simulink model "bbcSimPID"  (R2024a)
settings: Solver=VariableStepAuto  StartTime=0.0  StopTime=4.0  FixedStep=0.0001  RelTol=1e-3
model workspace (MAT data in the model file):
  V_ref = Simulink.Parameter
  V_ref.Complexity = 'real'
  V_ref.Dimensions = [0 0]
  V_ref.DataType = 'auto'
libraries: spsSeriesRLCBranchLib x3, spsVoltageMeasurementLib x2, spsDiodeLib x1, spsMosfetLib x1, spsDCVoltageSourceLib x1, spspowerguiLib x1, spsPWMGeneratorDCDCLib x1
settings Model: Creator=krupa  LastModifiedBy=ariellevy
settings OptimizationCC: ReuseModelBlockBuffer=off
settings RTWCC: GPUComputeCapability=3.5

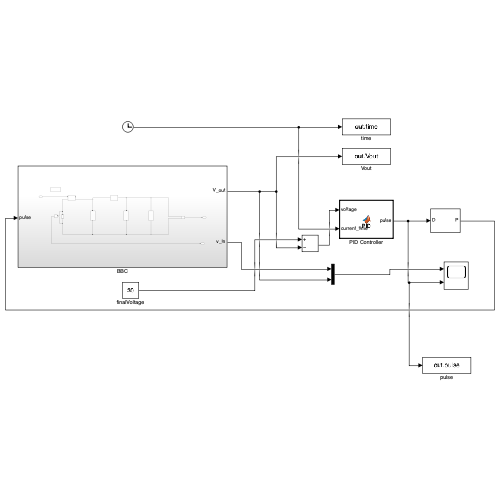
[thumbnail: Simulink's stored preview of the top-level diagram]
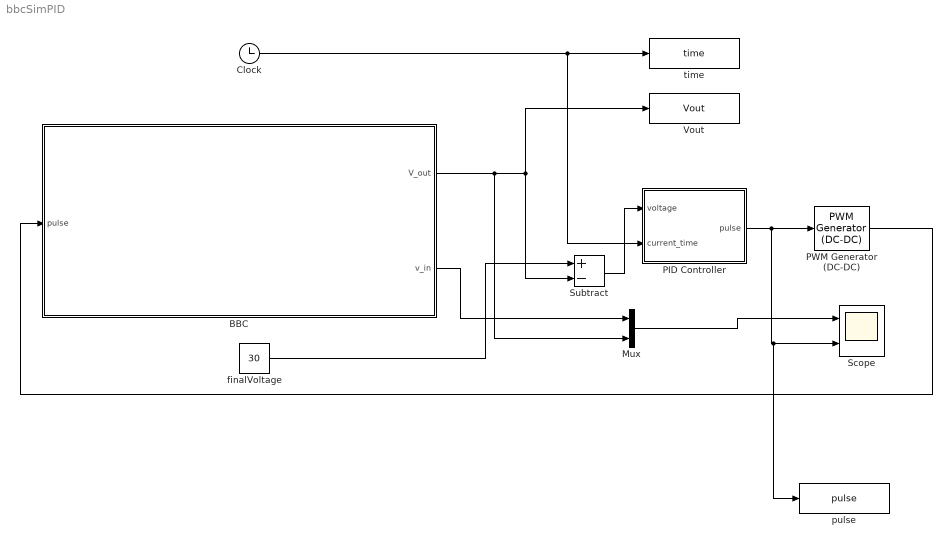
== system bbcSimPID ==
  BBC : Subsystem
  Clock : Clock
  Mux : Mux  Inputs=2
  PID Controller : MATLAB Function  TreatAsAtomicUnit=on  SystemSampleTime=0.0001
  PWM Generator (DC-DC) : spsPWMGeneratorDCDCLib/PWM Generator (DC-DC)  Fsw=10e3  Ts=0
  Scope : Scope  NumInputPorts=2
  Subtract : Sum  Inputs=+-
  Vout : ToWorkspace  VariableName=Vout  SampleTime=-1
  finalVoltage : Constant  Value=30
  pulse : ToWorkspace  VariableName=pulse  SampleTime=-1
  time : ToWorkspace  VariableName=time  SampleTime=-1
  wires:
  BBC/1(V_out) -> Mux/2, Subtract/2, Vout/1
  Clock/1 -> PID Controller/2(current_time), time/1
  PID Controller/1(pulse) -> pulse/1, Scope/2, PWM Generator (DC-DC)/1
  Subtract/1 -> PID Controller/1(voltage)
  finalVoltage/1 -> Subtract/1
  Mux/1 -> Scope/1
  BBC/2(v_in) -> Mux/1
  PWM Generator (DC-DC)/1 -> BBC/1(pulse)

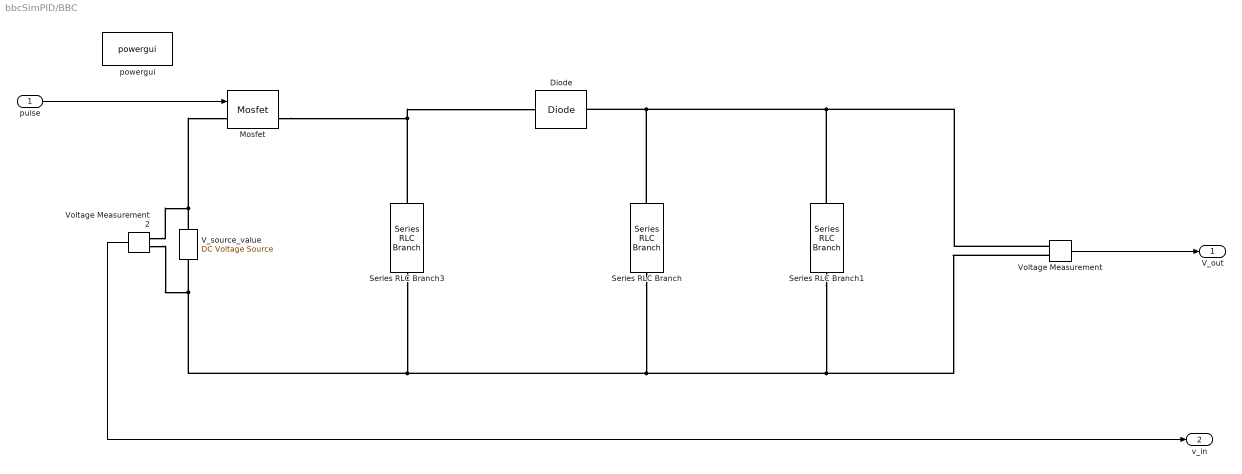
== system bbcSimPID/BBC ==
  pulse : Inport
  Diode : spsDiodeLib/Diode  Ron=0.001  Lon=0  Vf=0.8  IC=0  UseSnubber=0  Rs=500  Cs=250e-9  Measurements=off
  Mosfet : spsMosfetLib/Mosfet  Ron=0.1  Lon=0  Rd=0.01  Vfd=0  IC=0  Rs=1e5  Cs=inf  Measurements=on
  Series RLC Branch : spsSeriesRLCBranchLib/Series RLC Branch  LConnTagsString=__new0  RConnTagsString=__new0  BranchType=C  Resistance=1  Inductance=1e-3  SetiL0=off  InitialCurrent=0  Capacitance=40e-3  Setx0=off  InitialVoltage=0  Measurements=None
  Series RLC Branch1 : spsSeriesRLCBranchLib/Series RLC Branch  LConnTagsString=__new0  RConnTagsString=__new0  BranchType=R  Resistance=100  Inductance=1e-3  SetiL0=off  InitialCurrent=0  Capacitance=1e-6  Setx0=off  InitialVoltage=0  Measurements=None
  Series RLC Branch3 : spsSeriesRLCBranchLib/Series RLC Branch  LConnTagsString=__new0  RConnTagsString=__new0  BranchType=L  Resistance=1  Inductance=10e-6  SetiL0=off  InitialCurrent=0  Capacitance=1e-6  Setx0=off  InitialVoltage=0  Measurements=None
  V_source_value : spsDCVoltageSourceLib/DC Voltage Source  Amplitude=48  Measurements=Voltage
  Voltage Measurement : spsVoltageMeasurementLib/Voltage Measurement  PhasorSimulation=off  OutputType=Complex  PSBequivalent=0
  Voltage Measurement2 : spsVoltageMeasurementLib/Voltage Measurement  PhasorSimulation=off  OutputType=Complex  PSBequivalent=0
  powergui : spspowerguiLib/powergui  Priority=1  SimulationMode=Continuous  SampleTime=0.0001  frequency=60  Iterations=50  frequencyindice=0  Pbase=100e6  ErrMax=1e-4  UnitsV=kV  UnitsW=MW  buscounter=0  FunctionMessages=off  echomessages=off  EnableUseOfTLC=off  CurrentSourceSwitches=off  DisableSnubberDevices=off  DisableRonSwitches=off  DisableVfSwitches=off  DisplayEquations=off  AutomaticDiscreteSolvers=off  SolverType=Tustin/Backward Euler (TBE)  Interpol=off  ExternalGateDelay=off  methode=off  Ts=100  x0status=blocks  SPID=on  SwTol=0  HookPort=off  NonlinearTolerance=1e-4  nMaxIteration=100  ContinueOnMaxIteration=off  RestoreLinks=warning  ResistiveCurrentMeasurement=off  Frange=[0:2:500]  Ylog=off  Xlog=on  ShowGrid=off  save=off  variable=ZData  structure=0  ZoomFFT=off  StartTime=0.0  cycles=1  DisplayStyle=1  fundamental=60  FreqAxis=off  MaxFrequency=1000  frequencyindicesteady=1  RmsSteady=1  display=off
  V_out : Outport
  v_in : Outport  Port=2
  wires:
  pulse/1 -> Mosfet/1
  Voltage Measurement/1 -> V_out/1
  Voltage Measurement2/1 -> v_in/1
  connections:
  V_source_value/RConn1 -- Voltage Measurement2/LConn1 -- Mosfet/LConn1
  Mosfet/RConn1 -- Diode/RConn1 -- Series RLC Branch3/LConn1
  Voltage Measurement/LConn2 -- Series RLC Branch1/RConn1 -- Series RLC Branch/RConn1 -- Series RLC Branch3/RConn1 -- Voltage Measurement2/LConn2 -- V_source_value/LConn1
  Voltage Measurement/LConn1 -- Series RLC Branch1/LConn1 -- Series RLC Branch/LConn1 -- Diode/LConn1

== matlab function bbcSimPID/PID Controller ==
  settings: updateMethod=DISCRETE
  data: voltage input; pulse output; current_time input
function pulse = PID(voltage, current_time)

    % call extrinsic python function
    coder.extrinsic('py.PIDControllerBBC.controller_call');

    % Call Python function and return result
    pulse = coder.nullcopy(zeros(1,1)); % no clue why, but this is need.
    pulse = double(py.PIDControllerBBC.controller_call(voltage, current_time));
    end
